simulink subsystem "HardMon"  (R2023b)
settings: Solver=VariableStepAuto  StartTime=0.0  StopTime=10.0  RelTol=1e-3
libraries: simulink x3
settings Model: Creator=nickj  LastModifiedBy=diego

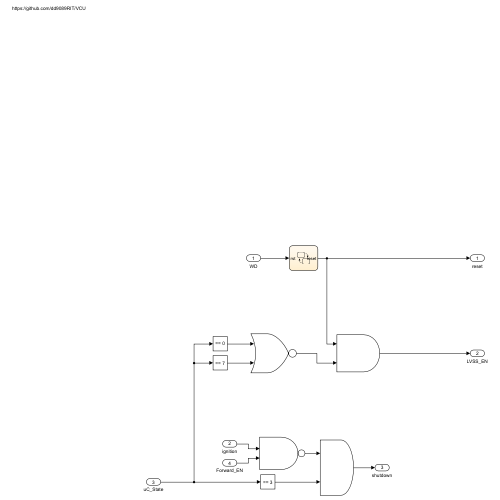
[thumbnail: Simulink's stored preview of the top-level diagram]
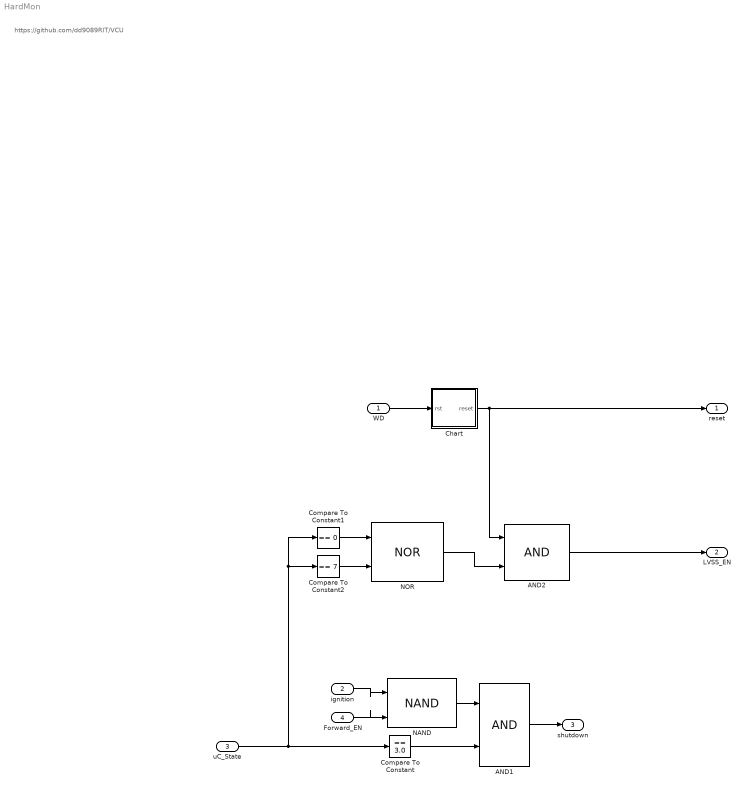
== system HardMon ==
  note: https://github.com/dd9089RIT/VCU
  WD : Inport
  ignition : Inport  Port=2
  uC_State : Inport  Port=3
  Forward_EN : Inport  Port=4
  AND1 : Logic  IconShape=distinctive  AllPortsSameDT=off  OutDataTypeStr=boolean
  AND2 : Logic  IconShape=distinctive  AllPortsSameDT=off  OutDataTypeStr=boolean
  Chart : Stateflow chart  TreatAsAtomicUnit=on
  Compare To Constant : simulink/Logic and Bit Operations/Compare To Constant  relop===  const=3.0  OutDataTypeStr=boolean
  Compare To Constant1 : simulink/Logic and Bit Operations/Compare To Constant  relop===  const=0  OutDataTypeStr=boolean
  Compare To Constant2 : simulink/Logic and Bit Operations/Compare To Constant  relop===  const=7  OutDataTypeStr=boolean
  NAND : Logic  Operator=NAND  IconShape=distinctive  AllPortsSameDT=off  OutDataTypeStr=boolean
  NOR : Logic  Operator=NOR  IconShape=distinctive  AllPortsSameDT=off  OutDataTypeStr=boolean
  reset : Outport
  LVSS_EN : Outport  Port=2
  shutdown : Outport  Port=3
  wires:
  uC_State/1 -> Compare To Constant1/1, Compare To Constant2/1, Compare To Constant/1
  ignition/1 -> NAND/1
  AND1/1 -> shutdown/1
  Compare To Constant/1 -> AND1/2
  NAND/1 -> AND1/1
  Forward_EN/1 -> NAND/2
  NOR/1 -> AND2/2
  Compare To Constant2/1 -> NOR/2
  Compare To Constant1/1 -> NOR/1
  AND2/1 -> LVSS_EN/1
  WD/1 -> Chart/1(rst)
  Chart/1(reset) -> reset/1, AND2/1

== stateflow chart HardMon/Chart ==
  state Normal
    entry:
    count = 0;
    state after
      entry:
      index = 0;
      (default) -> (junction 12) : % if
      (junction 12) -> (junction 13) [order 1] : [count == 4]
      (junction 12) -> (junction 14) [order 2]
      (junction 13) -> (junction 15) : {fault = 1;}
      (junction 15) -> (junction 14)
      (junction 14) -> (junction 16)
    state Default
      entry:
      index = 0;
    state Reset
      (default) -> (junction 65)
      (junction 65) -> (junction 74) [order 1] : [rst == 1]
      (junction 65) -> (junction 71) [order 2] : {count = count +1;}
      (junction 74) -> (junction 66) : {count = 0;}
      (junction 66) -> (junction 71)
      (junction 71) -> (junction 73) : {index = index +1;}
    (default) -> Default
    Default -> Reset : after(0.5,sec)
    Reset -> after [order 1] : [index == 4]
    after -> Reset
    Reset -> Reset [order 2] : after(0.5,sec)
  state Fault
    entry:
    reset = 1;
    on after(0.2,sec):
    reset = 0;
  (default) -> Normal
  Normal -> Fault : [fault == 1]
  data: fault local =0; rst input; count local; index local =0; reset output
